simulink model "simple_test_simulink1"  (Simulink 7.8)
settings: Solver=VariableStepDiscrete  StartTime=0.0  StopTime=0.0001  RelTol=1e-3
libraries: simulink x2
settings Model: Creator=labirint  LastModifiedBy=chuh
settings DebuggingCC: FcnCallInpInsideContextMsg=Use local settings  StrictBusMsg=Warning

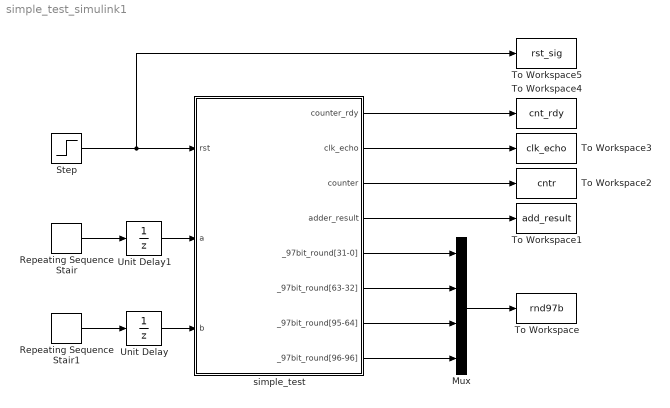
== system simple_test_simulink1 ==
  Mux : Mux
  Repeating Sequence Stair : simulink/Sources/Repeating Sequence Stair  OutValues=as_m  tsamp=1e-06  OutMin=[]  OutMax=[]  OutDataTypeStr=double  OutputDataTypeScalingMode=double  OutDataType=fixdt(0,8)  ConRadixGroup=Best Precision: Vector-wise  OutScaling=2^-12
  Repeating Sequence Stair1 : simulink/Sources/Repeating Sequence Stair  OutValues=bs_m  tsamp=1e-06  OutMin=[]  OutMax=[]  OutDataTypeStr=double  OutputDataTypeScalingMode=double  OutDataType=fixdt(0,8)  ConRadixGroup=Best Precision: Vector-wise  OutScaling=2^-12
  Step : Step  Time=5e-07  Before=1  After=0  SampleTime=0
  To Workspace : ToWorkspace  VariableName=rnd97b  SampleTime=5e-07  SaveFormat=Array
  To Workspace1 : ToWorkspace  VariableName=add_result  SampleTime=5e-07  SaveFormat=Array
  To Workspace2 : ToWorkspace  VariableName=cntr  SampleTime=5e-07  SaveFormat=Array
  To Workspace3 : ToWorkspace  VariableName=clk_echo  SampleTime=5e-07  SaveFormat=Array
  To Workspace4 : ToWorkspace  VariableName=cnt_rdy  SampleTime=5e-07  SaveFormat=Array
  To Workspace5 : ToWorkspace  VariableName=rst_sig  SampleTime=5e-07  SaveFormat=Structure With Time
  Unit Delay : UnitDelay  SampleTime=1e-06
  Unit Delay1 : UnitDelay  SampleTime=1e-06
  simple_test : Subsystem  mask(simple_test){params_samples=5e-07, params_freq=1}
      mask prompts: params_samples "Sample time:"; params_freq "FPGA frequency (MHz):"
      mask help:
      | input rst
      | input a[30:0]
      | input b[30:0]
      | output counter_rdy
      | output clk_echo
      | output counter[15:0]
      | output adder_result[31:0]
      | output _97bit_round[96:0]
      mask Help:
      | input rst
      | input a[30:0]
      | input b[30:0]
      | output counter_rdy
      | output clk_echo
      | output counter[15:0]
      | output adder_result[31:0]
      | output _97bit_round[96:0]
  wires:
  Step/1 -> simple_test/1(rst), To Workspace5/1
  Repeating Sequence Stair/1 -> Unit Delay1/1
  Repeating Sequence Stair1/1 -> Unit Delay/1
  simple_test/5(_97bit_round[31-0]) -> Mux/1
  simple_test/6(_97bit_round[63-32]) -> Mux/2
  simple_test/7(_97bit_round[95-64]) -> Mux/3
  simple_test/8(_97bit_round[96-96]) -> Mux/4
  Mux/1 -> To Workspace/1
  simple_test/4(adder_result) -> To Workspace1/1
  simple_test/3(counter) -> To Workspace2/1
  simple_test/2(clk_echo) -> To Workspace3/1
  simple_test/1(counter_rdy) -> To Workspace4/1
  Unit Delay/1 -> simple_test/3(b)
  Unit Delay1/1 -> simple_test/2(a)

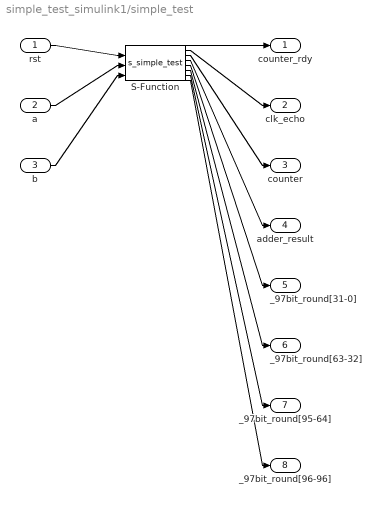
== system simple_test_simulink1/simple_test ==
  rst : Inport  OutDataTypeStr=double  SampleTime=5e-07
  a : Inport  Port=2  OutDataTypeStr=double  SampleTime=5e-07
  b : Inport  Port=3  OutDataTypeStr=double  SampleTime=5e-07
  S-Function : S-Function  FunctionName=s_simple_test  Parameters=params_samples, params_freq  EnableBusSupport=off
  counter_rdy : Outport  OutDataTypeStr=uint32  SampleTime=5e-07
  clk_echo : Outport  Port=2  OutDataTypeStr=uint32  SampleTime=5e-07
  counter : Outport  Port=3  OutDataTypeStr=uint32  SampleTime=5e-07
  adder_result : Outport  Port=4  OutDataTypeStr=uint32  SampleTime=5e-07
  _97bit_round[31-0] : Outport  Port=5  OutDataTypeStr=uint32  SampleTime=5e-07
  _97bit_round[63-32] : Outport  Port=6  OutDataTypeStr=uint32  SampleTime=5e-07
  _97bit_round[95-64] : Outport  Port=7  OutDataTypeStr=uint32  SampleTime=5e-07
  _97bit_round[96-96] : Outport  Port=8  OutDataTypeStr=uint32  SampleTime=5e-07
  wires:
  rst/1 -> S-Function/1
  a/1 -> S-Function/2
  b/1 -> S-Function/3
  S-Function/1 -> counter_rdy/1
  S-Function/2 -> clk_echo/1
  S-Function/3 -> counter/1
  S-Function/4 -> adder_result/1
  S-Function/5 -> _97bit_round[31-0]/1
  S-Function/6 -> _97bit_round[63-32]/1
  S-Function/7 -> _97bit_round[95-64]/1
  S-Function/8 -> _97bit_round[96-96]/1
